simulink model "benchmark_16bus_base_scenario"  (R2021a)
settings: Solver=ode4  StartTime=0.0  StopTime=5  FixedStep=Ts  MaxStep=50e-6  RelTol=1e-3
values from neighbouring files (symbols this model uses):
  Ctrl_Delay = 100e-6    (= 0.0001)    [init_anon.m]
  Pnom1 = 1330e6    (= 1330000000)    [init_anon.m]
  Pnom3 = 1e9    (= 1000000000)    [init_anon.m]
  Pnom4 = 64.4e6    (= 64400000)    [init_anon.m]
  Pnom5 = 19e6    (= 19000000)    [init_anon.m]
  Pnom6 = 450e6    (= 450000000)    [init_anon.m]
  Snom1 = 1e6*sqrt(1330^2 + (0.3*1330)^2)    [init_anon.m]
  Snom3 = 1044e6    (= 1044000000)    [init_anon.m]
  Snom4 = 1e6*sqrt(64.4^2 + (0.3*64.4)^2)    [init_anon.m]
  Snom5 = 1e6*sqrt(19^2 + (0.3*19)^2)    [init_anon.m]
  Snom6 = 1e6*sqrt(450^2 + (0.3*450)^2)    [init_anon.m]
  Ts = 5e-6    (= 5e-06)    [init_anon.m]
  wb = 2*pi*50    (= 314.159265359)    [init_anon.m]
  wcc = 1200    [init_anon.m]
  wlpf = 300    [init_anon.m]
  wp = 10    [init_anon.m]
  wv = 50    [init_anon.m]
  Zb = Ub^2/Sb    [init_anon.m]
undefined symbols (not defined in the file or in its folder): fb, Ib2, Ki_CC, Ki_i, Kp_CC, Kp_i, Kp_Rvi_pu, Lc_eq, Lf_pu, Rc_eq, Sb, Va0, Vb0, Vb1, Vb2, Vc0, Vm0, Vm0_d, Vm0_q, VSC01_id0, Vvsc0
libraries: spsGroundLib x135, spsParallelRLCBranchLib x132, Control_Lib x120, spsSeriesRLCBranchLib x66, spsThreePhaseSourceLib x22, spsThreePhaseBreakerLib x20, eeGeneralControl x20, slpidlib x15, spsLoadFlowBusLib x13, spsThreePhaseVIMeasurementLib x12, spsThreePhaseTransformerTwoWindingsLib x11, spsUniversalBridgeLib x10
(part 5 of 9)

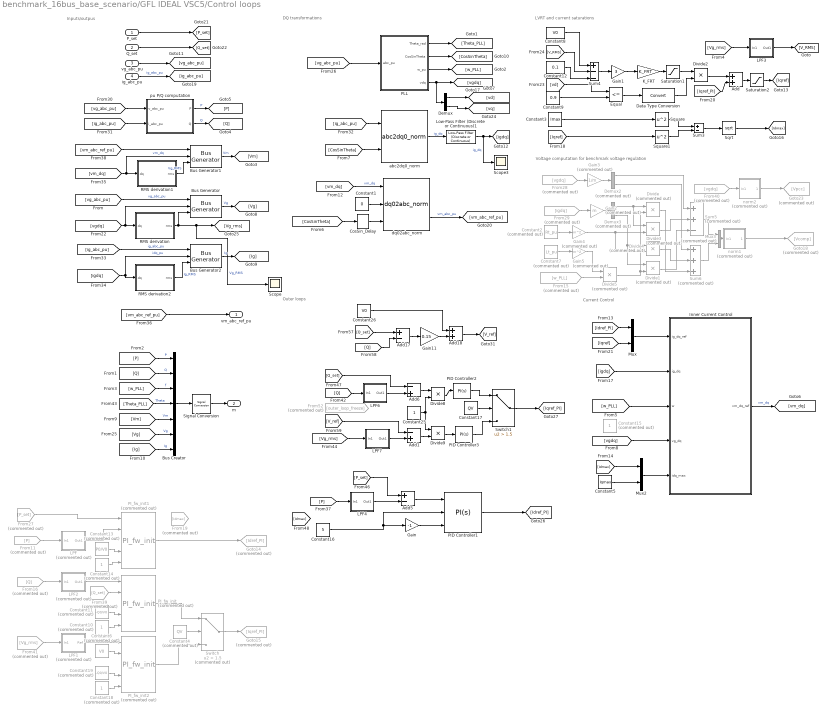
== system benchmark_16bus_base_scenario/GFL IDEAL VSC5/Control loops ==
  note: Inputs/outpus
  note: DQ transformations
  note: Current Control
  note: Outer loops
  note: LVRT and current saturations
  note: Voltage computation for benchmark voltage regulation
  P_set : Inport
  Q_set : Inport  Port=2
  vg_abc_pu : Inport  Port=3
  ig_abc_pu : Inport  Port=4
  " pu P/Q computation" : Subsystem  DialogController=POWERSYS.PowerSysDialog
  Add : Sum
  Add1 : Sum  Inputs=-+
  Add17 : Sum  Inputs=+-
  Add18 : Sum
  Add5 : Sum  Inputs=+-
  Add6 : Sum  Inputs=-+
  Bus Creator : BusCreator  Inputs=7
  Bus Generator : Control_Lib/Bus Generator  Gpu=0
      settings: SourceProductName=VSC4SPS
  Bus Generator1 : Control_Lib/Bus Generator  Gpu=0
      settings: SourceProductName=VSC4SPS
  Bus Generator2 : Control_Lib/Bus Generator  Gpu=0
      settings: SourceProductName=VSC4SPS
  Constant1 : Constant  Value=0
  Constant{10,14..15,18} (4 alike) : Constant  Commented=on
  Constant11 : Constant  Commented=on  Value=-Q0/V0
  Constant12 : Constant  Value=0.1
  Constant13 : Constant  Commented=on  Value=P0/V0
  Constant16 : Constant  Value=5
  Constant17 : Constant  Value=QV
  Constant19 : Constant  Commented=on  Value=-Q0/V0
  Constant2 : Constant  Commented=on  Value=Rt_pu
  Constant25 : Constant
  Constant26 : Constant  Value=V0
  Constant3 : Constant  Value=Imax
  Constant4 : Constant  Commented=on  Value=QV
  Constant5 : Constant  Value=Iqmax
  Constant6 : Constant  Commented=on  Value=V0
  Constant7 : Constant  Commented=on  Value=Lt_pu
  Constant8 : Constant  Value=V0
  Constant9 : Constant  Value=0.9
  CosSin_Delay : Control_Lib/CosSin_Delay  dTheta=wb*Output_Delay
      settings: SourceProductName=VSC4SPS
  Data Type Conversion : DataTypeConversion
  Demux : Demux  Outputs=[1 1]
  Demux2 : Demux  Commented=on  Outputs=2
  Demux3 : Demux  Commented=on  Outputs=2
  Divide{,1,3..5} (5 alike) : Product  Commented=on  Inputs=**
  Divide2 : Product  Inputs=**
  Divide8 : Product  Inputs=**
  Divide9 : Product  Inputs=**
  Equal : RelationalOperator  Operator=<=  OutDataTypeStr=boolean  RndMeth=Simplest
  From11 : From  Commented=on  GotoTag=P
  From15 : From  Commented=on  GotoTag=w_PLL
  From16 : From  Commented=on  GotoTag=Q
  From19 : From  Commented=on  GotoTag=Idmax
  From27 : From  Commented=on  GotoTag=P_set
  From28 : From  Commented=on  GotoTag=vgdq
  From29 : From  Commented=on  GotoTag=igdq
  From39 : From  Commented=on  GotoTag=Q_set
  From40 : From  Commented=on  GotoTag=vgdq
  From41 : From  Commented=on  GotoTag=Vg_rms
  From52 : From  Commented=on  GotoTag=outer_loop_freeze
  Gain : Gain  Gain=-1
  Gain1 : Gain  Gain=3
  Gain11 : Gain  Gain=0.15
  Gain2 : Gain  Commented=on  Gain=m
  Gain3 : Gain  Commented=on  Gain=1/m
  Gain4 : Gain  Commented=on  Gain=m^2
  Gain5 : Gain  Commented=on  Gain=m^2
  Goto14 : Goto  Commented=on  GotoTag=Idref_PI
  Goto15 : Goto  Commented=on  GotoTag=Iqref_PI
  Goto18 : Goto  Commented=on  GotoTag=Vcomp
  Goto23 : Goto  Commented=on  GotoTag=Vpcc
  Inner Current Control : Subsystem
  K_FRT : Gain  Gain=K_FRT
  LPF : Subsystem  Commented=on
  LPF1 : Subsystem  Commented=on
  LPF2 : Subsystem  Commented=on
  LPF3 : Subsystem
  LPF4 : Subsystem
  LPF6 : Subsystem
  LPF7 : Subsystem
  Low-Pass Filter (Discrete or Continuous)1 : eeGeneralControl/Low-Pass Filter (Discrete or Continuous)  K=1  T=1/(2*pi*1e4)  B=inf  A=-inf  init_option=Specify as parameter  x0=[P0/V0 -Q0/V0]  Ts=-1
  Mux : Mux  Inputs=2
  Mux2 : Mux  Inputs=2
  Mux3 : Mux  Commented=on  Inputs=2
  PID Controller1 : slpidlib/PID Controller  Controller=PI  Form=Parallel  TimeDomain=Continuous-time  UseExternalTs=off  SampleTime=-1  IntegratorMethod=Forward Euler  FilterMethod=Forward Euler  ControllerParametersSource=internal  P=w_P/w_LPF  I=w_P  D=0  UseFilter=on  N=100  TunerSelectOption=Transfer Function Based (PID Tuner App)  InitialConditionSource=internal  InitialConditionForIntegrator=P0/V0  InitialConditionForFilter=0  DifferentiatorICPrevScaledInput=0  ExternalReset=none  TrackingMode=off  Kt=1  LimitOutput=on  SatLimitsSource=external  UpperSaturationLimit=inf  LowerSaturationLimit=-inf  LinearizeAsGain=on  AntiWindupMode=clamping  Kb=1  POutMin=[]  POutMax=[]  IOutMin=[]  IOutMax=[]  DOutMin=[]  DOutMax=[]  NOutMin=[]  NOutMax=[]  SumOutMin=[]  SumOutMax=[]  SaturationOutMin=[]  SaturationOutMax=[]  PParamMin=[]  PParamMax=[]  IParamMin=[]  IParamMax=[]  DParamMin=[]  DParamMax=[]  NParamMin=[]  NParamMax=[]  KbParamMin=[]  KbParamMax=[]  KtParamMin=[]  KtParamMax=[]  KbOutMin=[]  KbOutMax=[]  KtOutMin=[]  KtOutMax=[]  IntegratorOutMin=[]  IntegratorOutMax=[]  FilterOutMin=[]  FilterOutMax=[]  SumI1OutMin=[]  SumI1OutMax=[]  SumI2OutMin=[]  SumI2OutMax=[]  SumI3OutMin=[]  SumI3OutMax=[]  SumI4OutMin=[]  SumI4OutMax=[]  SumDOutMin=[]  SumDOutMax=[]  DifferentiatorOutMin=[]  DifferentiatorOutMax=[]  FilterDiffOutCoefMin=[]  FilterDiffOutCoefMax=[]  ReciprocalOutMin=[]  ReciprocalOutMax=[]  SumDenOutMin=[]  SumDenOutMax=[]  SumNumOutMin=[]  SumNumOutMax=[]  DivideOutMin=[]  DivideOutMax=[]  UdiffTsProdOutMin=[]  UdiffTsProdOutMax=[]  NTsProdOutMin=[]  NTsProdOutMax=[]  UintegralTsProdOutMin=[]  UintegralTsProdOutMax=[]  UngainTsProdOutMin=[]  UngainTsProdOutMax=[]  IntegratorContinuousStateAttributes=''  IntegratorStateMustResolveToSignalObject=off  IntegratorRTWStateStorageClass=Auto  FilterContinuousStateAttributes=''  FilterStateMustResolveToSignalObject=off  FilterRTWStateStorageClass=Auto  ParallelPVariant=InternalParameters  IdealPVariant=Disabled  IVariant=InternalParameters  DVariant=Disabled  IntegratorVariant=Continuous  SatVariant=External  AWVariant=ContClampingParallel  PCopyVariant=Disabled  TRVariant=Disabled  FdbkBlocksVariant=Forward  IdealPFdbkVariant=Disabled  SatFdbkVariant=Disabled  DerivativeFilterVariant=Disabled  NVariant=Disabled  NCopyVariant=Disabled_SignalSpec  FilterICVariant=Disabled  IntegratorICVariant=InternalICs  ExternalResetVariant=Disabled  TRSumVariant=Passthrough  SumFdbkVariant=Disabled  SumVariant=Sum_PI  TsampFilterVariant=InternalTs  TsampNgainVariant=Passthrough  TsampIntegralVariant=Passthrough  ExternalSaturationOutDataTypeStr=Inherit: Same as second input
  PID Controller2 : slpidlib/PID Controller  Controller=PI  Form=Parallel  TimeDomain=Continuous-time  UseExternalTs=off  SampleTime=-1  IntegratorMethod=Forward Euler  FilterMethod=Forward Euler  ControllerParametersSource=internal  P=w_P/w_LPF  I=w_P  D=0  UseFilter=on  N=100  TunerSelectOption=Transfer Function Based (PID Tuner App)  InitialConditionSource=internal  InitialConditionForIntegrator=-Q0/V0  InitialConditionForFilter=0  DifferentiatorICPrevScaledInput=0  ExternalReset=none  TrackingMode=off  Kt=1  LimitOutput=on  SatLimitsSource=internal  UpperSaturationLimit=Iqmax*m  LowerSaturationLimit=-Iqmax*m  LinearizeAsGain=on  AntiWindupMode=clamping  Kb=1  POutMin=[]  POutMax=[]  IOutMin=[]  IOutMax=[]  DOutMin=[]  DOutMax=[]  NOutMin=[]  NOutMax=[]  SumOutMin=[]  SumOutMax=[]  SaturationOutMin=[]  SaturationOutMax=[]  PParamMin=[]  PParamMax=[]  IParamMin=[]  IParamMax=[]  DParamMin=[]  DParamMax=[]  NParamMin=[]  NParamMax=[]  KbParamMin=[]  KbParamMax=[]  KtParamMin=[]  KtParamMax=[]  KbOutMin=[]  KbOutMax=[]  KtOutMin=[]  KtOutMax=[]  IntegratorOutMin=[]  IntegratorOutMax=[]  FilterOutMin=[]  FilterOutMax=[]  SumI1OutMin=[]  SumI1OutMax=[]  SumI2OutMin=[]  SumI2OutMax=[]  SumI3OutMin=[]  SumI3OutMax=[]  SumI4OutMin=[]  SumI4OutMax=[]  SumDOutMin=[]  SumDOutMax=[]  DifferentiatorOutMin=[]  DifferentiatorOutMax=[]  FilterDiffOutCoefMin=[]  FilterDiffOutCoefMax=[]  ReciprocalOutMin=[]  ReciprocalOutMax=[]  SumDenOutMin=[]  SumDenOutMax=[]  SumNumOutMin=[]  SumNumOutMax=[]  DivideOutMin=[]  DivideOutMax=[]  UdiffTsProdOutMin=[]  UdiffTsProdOutMax=[]  NTsProdOutMin=[]  NTsProdOutMax=[]  UintegralTsProdOutMin=[]  UintegralTsProdOutMax=[]  UngainTsProdOutMin=[]  UngainTsProdOutMax=[]  IntegratorContinuousStateAttributes=''  IntegratorStateMustResolveToSignalObject=off  IntegratorRTWStateStorageClass=Auto  FilterContinuousStateAttributes=''  FilterStateMustResolveToSignalObject=off  FilterRTWStateStorageClass=Auto  ParallelPVariant=InternalParameters  IdealPVariant=Disabled  IVariant=InternalParameters  DVariant=Disabled  IntegratorVariant=Continuous  SatVariant=Enabled  AWVariant=ContClampingParallel  PCopyVariant=Disabled  TRVariant=Disabled  FdbkBlocksVariant=Forward  IdealPFdbkVariant=Disabled  SatFdbkVariant=Disabled  DerivativeFilterVariant=Disabled  NVariant=Disabled  NCopyVariant=Disabled_SignalSpec  FilterICVariant=Disabled  IntegratorICVariant=InternalICs  ExternalResetVariant=Disabled  TRSumVariant=Passthrough  SumFdbkVariant=Disabled  SumVariant=Sum_PI  TsampFilterVariant=InternalTs  TsampNgainVariant=Passthrough  TsampIntegralVariant=Passthrough  ExternalSaturationOutDataTypeStr=Inherit: Same as second input
  PID Controller3 : slpidlib/PID Controller  Controller=PI  Form=Parallel  TimeDomain=Continuous-time  UseExternalTs=off  SampleTime=-1  IntegratorMethod=Forward Euler  FilterMethod=Forward Euler  ControllerParametersSource=internal  P=w_V/w_LPF  I=w_V  D=0  UseFilter=on  N=100  TunerSelectOption=Transfer Function Based (PID Tuner App)  InitialConditionSource=internal  InitialConditionForIntegrator=-Q0/V0  InitialConditionForFilter=0  DifferentiatorICPrevScaledInput=0  ExternalReset=none  TrackingMode=off  Kt=1  LimitOutput=on  SatLimitsSource=internal  UpperSaturationLimit=Iqmax*m  LowerSaturationLimit=-Iqmax*m  LinearizeAsGain=on  AntiWindupMode=clamping  Kb=1  POutMin=[]  POutMax=[]  IOutMin=[]  IOutMax=[]  DOutMin=[]  DOutMax=[]  NOutMin=[]  NOutMax=[]  SumOutMin=[]  SumOutMax=[]  SaturationOutMin=[]  SaturationOutMax=[]  PParamMin=[]  PParamMax=[]  IParamMin=[]  IParamMax=[]  DParamMin=[]  DParamMax=[]  NParamMin=[]  NParamMax=[]  KbParamMin=[]  KbParamMax=[]  KtParamMin=[]  KtParamMax=[]  KbOutMin=[]  KbOutMax=[]  KtOutMin=[]  KtOutMax=[]  IntegratorOutMin=[]  IntegratorOutMax=[]  FilterOutMin=[]  FilterOutMax=[]  SumI1OutMin=[]  SumI1OutMax=[]  SumI2OutMin=[]  SumI2OutMax=[]  SumI3OutMin=[]  SumI3OutMax=[]  SumI4OutMin=[]  SumI4OutMax=[]  SumDOutMin=[]  SumDOutMax=[]  DifferentiatorOutMin=[]  DifferentiatorOutMax=[]  FilterDiffOutCoefMin=[]  FilterDiffOutCoefMax=[]  ReciprocalOutMin=[]  ReciprocalOutMax=[]  SumDenOutMin=[]  SumDenOutMax=[]  SumNumOutMin=[]  SumNumOutMax=[]  DivideOutMin=[]  DivideOutMax=[]  UdiffTsProdOutMin=[]  UdiffTsProdOutMax=[]  NTsProdOutMin=[]  NTsProdOutMax=[]  UintegralTsProdOutMin=[]  UintegralTsProdOutMax=[]  UngainTsProdOutMin=[]  UngainTsProdOutMax=[]  IntegratorContinuousStateAttributes=''  IntegratorStateMustResolveToSignalObject=off  IntegratorRTWStateStorageClass=Auto  FilterContinuousStateAttributes=''  FilterStateMustResolveToSignalObject=off  FilterRTWStateStorageClass=Auto  ParallelPVariant=InternalParameters  IdealPVariant=Disabled  IVariant=InternalParameters  DVariant=Disabled  IntegratorVariant=Continuous  SatVariant=Enabled  AWVariant=ContClampingParallel  PCopyVariant=Disabled  TRVariant=Disabled  FdbkBlocksVariant=Forward  IdealPFdbkVariant=Disabled  SatFdbkVariant=Disabled  DerivativeFilterVariant=Disabled  NVariant=Disabled  NCopyVariant=Disabled_SignalSpec  FilterICVariant=Disabled  IntegratorICVariant=InternalICs  ExternalResetVariant=Disabled  TRSumVariant=Passthrough  SumFdbkVariant=Disabled  SumVariant=Sum_PI  TsampFilterVariant=InternalTs  TsampNgainVariant=Passthrough  TsampIntegralVariant=Passthrough  ExternalSaturationOutDataTypeStr=Inherit: Same as second input
  PI_fw_init : Control_Lib/PI_fw_init  Commented=on  Kp=w_P/w_LPF  Ki=w_P
      settings: SourceProductName=VSC4SPS
  PI_fw_init1 : Control_Lib/PI_fw_init  Commented=on  Kp=w_P/w_LPF  Ki=w_P
      settings: SourceProductName=VSC4SPS
  PI_fw_init2 : Control_Lib/PI_fw_init  Commented=on  Kp=w_V/w_LPF  Ki=w_V
      settings: SourceProductName=VSC4SPS
  PLL : Subsystem  AncestorBlock=Control_Lib/PLL  TreatAsAtomicUnit=on  mask{fb=fb, wn_PLL=wn_PLL, zeta_PLL=zeta_PLL, Theta0=Theta0}
      mask prompts: fb "fb (Hz)"; wn_PLL "Bandwidth (rad/s)"; zeta_PLL "Damping Ratio"; Theta0 "Theta0 (°)"
      mask init:
      | wb = 2*pi*fb;
      | Kp_PLL = 2*zeta_PLL*wn_PLL/wb;
      | Ki_PLL = wn_PLL^2/wb;
  RMS derivation : Subsystem
  RMS derivation1 : Subsystem
  RMS derivation2 : Subsystem
  Saturation1 : Saturate  UpperLimit=Imax  LowerLimit=-Imax
  Saturation2 : Saturate  UpperLimit=Imax  LowerLimit=-Imax
  Scope : Scope
  Scope3 : Scope
  Signal Conversion : SignalConversion  OverrideOpt=off
  Sqrt : Sqrt  SaturateOnIntegerOverflow=on
  Square : Math  Operator=square  SaturateOnIntegerOverflow=on
  Square1 : Math  Operator=square  SaturateOnIntegerOverflow=on
  Sum3 : Sum  Inputs=+-
  Sum4 : Sum  Inputs=+--
  Sum5 : Sum  Commented=on  Inputs=++-
  Sum6 : Sum  Commented=on  Inputs=+++
  Switch : Switch  Commented=on  Criteria=u2 > Threshold  Threshold=1.5
  Switch1 : Switch  Criteria=u2 > Threshold  Threshold=1.5
  abc2dq0_norm : Control_Lib/abc2dq0_norm  referenceAxisMode=Reference axis at 90 degrees behind phase_a  baseUpdateGain=1/sqrt(3)
      settings: SourceProductName=VSC4SPS
  dq02abc_norm : Control_Lib/dq02abc_norm  referenceAxisMode=Reference axis at 90 degrees behind phase_a  baseUpdateGain=sqrt(3)
      settings: SourceProductName=VSC4SPS
  norm1 : Subsystem  Commented=on
  norm2 : Subsystem  Commented=on
  vm_abc_ref_pu : Outport  VectorParamsAs1DForOutWhenUnconnected=off
  m : Outport  Port=2  VectorParamsAs1DForOutWhenUnconnected=off
  wires:
  Low-Pass Filter (Discrete or Continuous)1/1 -> Scope3/1, [igdq]  "ig_dq"
  [Q_set] -> Add6/1
  [P_set] -> Add5/1
  Switch1/1 -> [Iqref_PI]
  Gain/1 -> PID Controller1/3
  PID Controller3/1 -> Switch1/3
  [Vg_rms] -> LPF7/1(In1)
  PID Controller2/1 -> Switch1/1
  [Q] -> LPF6/1(In1)
  Constant17/1 -> Switch1/2
  Add5/1 -> PID Controller1/1
  LPF4/1(Out1) -> Add5/2
  [P] -> LPF4/1(In1)
  LPF6/1(Out1) -> Add6/2
  PID Controller1/1 -> [Idref_PI]
  Add6/1 -> Divide8/1
  Divide8/1 -> PID Controller2/1
  Divide9/1 -> PID Controller3/1
  Add1/1 -> Divide9/2
  Constant25/1 -> Divide9/1, Divide8/2
  Constant16/1 -> Gain/1, PID Controller1/2
  LPF7/1(Out1) -> Add1/2
  [V_ref] -> Add1/1
  [Q] -> Add17/2
  Constant26/1 -> Add18/1
  [Q_set] -> Add17/1
  Gain11/1 -> Add18/2
  Add17/1 -> Gain11/1
  Add18/1 -> [V_ref]
  [w_PLL] -> Inner Current Control/3(w)
  Constant6/1 -> PI_fw_init2/2
  PI_fw_init2/1 -> Switch/3
  Constant14/1 -> PI_fw_init1/5
  Constant13/1 -> PI_fw_init1/4
  [Vg_rms] -> LPF3/1(In1)
  LPF3/1(Out1) -> [V_RMS]
  CosSin_Delay/1 -> dq02abc_norm/3
  [Theta_PLL] -> Bus Creator/4  "Theta"
  RMS derivation/1(rms) -> Bus Generator/3, [Vg_rms], Scope/1  "Vg_RMS"
  [vgdq] -> Bus Generator/2, RMS derivation/1(dq)
  Demux/2 -> [vq]
  Demux/1 -> [vd]
  PLL/4(vdq) -> [vgdq], Demux/1
  norm2/1(Out1) -> Goto23/1
  From40/1 -> norm2/1(In1)
  Gain4/1 -> Divide3/2, Divide4/2
  Gain5/1 -> Divide5/1
  Gain2/1 -> Demux3/1
  From29/1 -> Gain2/1
  From39/1 -> PI_fw_init/2
  [vgdq] -> Inner Current Control/4(vg_dq)
  [vm_abc_ref_pu] -> Bus Generator1/1
  [vm_abc_ref_pu] -> vm_abc_ref_pu/1
  [vm_dq] -> Bus Generator1/2, RMS derivation1/1(dq)  "vm_dq"
  [ig_abc_pu] -> abc2dq0_norm/1
  [ig_abc_pu] -> " pu P/Q computation"/2(i_abc_pu)
  [vg_abc_pu] -> " pu P/Q computation"/1(v_abc_pu)
  [vg_abc_pu] -> PLL/1(abc_pu)
  From41/1 -> LPF1/1(In1)
  Constant7/1 -> Gain5/1
  From15/1 -> Divide5/2
  PLL/3(w_pu) -> [w_PLL]
  PLL/2(CosSinTheta) -> [CosSinTheta]
  PLL/1(Theta_rad) -> [Theta_PLL]
  Demux3/1 -> Divide3/1, Divide/1
  Divide4/1 -> Sum6/2
  Demux3/2 -> Divide4/1, Divide1/1
  Divide3/1 -> Sum5/2
  Demux2/1 -> Sum5/1
  Divide5/1 -> Divide1/2, Divide/2
  Divide/1 -> Sum6/3
  Mux3/1 -> norm1/1(In1)
  Sum6/1 -> Mux3/2
  Divide1/1 -> Sum5/3
  norm1/1(Out1) -> Goto18/1
  Constant2/1 -> Gain4/1
  Gain3/1 -> Demux2/1
  Demux2/2 -> Sum6/1
  From28/1 -> Gain3/1
  Sum5/1 -> Mux3/1
  Gain1/1 -> K_FRT/1
  [Iqref] -> Square1/1
  Square/1 -> Sum3/1
  Constant3/1 -> Square/1
  Sum3/1 -> Sqrt/1
  Sqrt/1 -> [Idmax]
  Square1/1 -> Sum3/2
  LPF1/1(Ref) -> PI_fw_init2/1
  Q_set/1 -> [Q_set]
  From16/1 -> LPF2/1(In1)
  [Idmax] -> Mux2/1
  Constant5/1 -> Mux2/2
  Mux2/1 -> Inner Current Control/5(idq_max)
  [Iqref_PI] -> Add/2
  Add/1 -> Saturation2/1
  Constant4/1 -> Switch/2
  Constant9/1 -> Equal/2
  Constant8/1 -> Sum4/1
  Constant12/1 -> Sum4/3
  Divide2/1 -> Add/1
  [vd] -> Equal/1
  Data Type Conversion/1 -> Divide2/2
  Equal/1 -> Data Type Conversion/1
  Saturation1/1 -> Divide2/1
  K_FRT/1 -> Saturation1/1
  [V_RMS] -> Sum4/2
  Sum4/1 -> Gain1/1
  Saturation2/1 -> [Iqref]
  [igdq] -> Inner Current Control/2(ig_dq)
  [Idref_PI] -> Mux/1
  [Iqref] -> Mux/2
  From11/1 -> LPF/1(In1)
  P_set/1 -> [P_set]
  Bus Creator/1 -> Signal Conversion/1
  Bus Generator/1 -> [Vg]  "Vg"
  [CosSinTheta] -> abc2dq0_norm/2
  [CosSinTheta] -> CosSin_Delay/1
  abc2dq0_norm/2 -> Low-Pass Filter (Discrete or Continuous)1/1  "ig_dq"
  ig_abc_pu/1 -> [ig_abc_pu]  "ig_abc_pu"
  " pu P/Q computation"/1(P) -> [P]  "P"
  vg_abc_pu/1 -> [vg_abc_pu]
  Inner Current Control/1(vm_dq_ref) -> [vm_dq]  "vm_dq"
  [vm_dq] -> dq02abc_norm/1  "vm_dq"
  " pu P/Q computation"/2(Q) -> [Q]  "Q"
  dq02abc_norm/2 -> [vm_abc_ref_pu]  "vm_abc_pu"
  [w_PLL] -> Bus Creator/3  "f"
  [Q] -> Bus Creator/2  "Q"
  [P] -> Bus Creator/1  "P"
  Signal Conversion/1 -> m/1
  Mux/1 -> Inner Current Control/1(ig_dq_ref)
  Constant1/1 -> dq02abc_norm/2
  [vg_abc_pu] -> Bus Generator/1  "vg_abc_pu"
  RMS derivation1/1(rms) -> Bus Generator1/3  "Vg_RMS"
  Bus Generator1/1 -> [Vm]  "Vm"
  [Vm] -> Bus Creator/5  "Vm"
  [Vg] -> Bus Creator/6  "Vg"
  [Ig] -> Bus Creator/7  "Ig"
  [ig_abc_pu] -> Bus Generator2/1  "ig_abc_pu"
  Bus Generator2/1 -> [Ig]  "Ig"
  [igdq] -> RMS derivation2/1(dq), Bus Generator2/2  "idq_pu"
  RMS derivation2/1(rms) -> Bus Generator2/3  "Ig_RMS"
  Constant11/1 -> PI_fw_init/4
  Constant10/1 -> PI_fw_init/5
  PI_fw_init/1 -> Switch/1
  LPF2/1(Out1) -> PI_fw_init/1
  Constant18/1 -> PI_fw_init2/5
  Constant19/1 -> PI_fw_init2/4
  Switch/1 -> Goto15/1
  LPF/1(Out1) -> PI_fw_init1/2
  From27/1 -> PI_fw_init1/1
  PI_fw_init1/1 -> Goto14/1

== system benchmark_16bus_base_scenario/GFL IDEAL VSC6/Bridge_Model ==
  Uref : Inport
  NOT1 : Logic  Operator=NOT  IconShape=distinctive  AllPortsSameDT=off  OutDataTypeStr=boolean
  Saturation : Saturate  UpperLimit=1  LowerLimit=-1
  Step : Step  Time=Output_Delay  SampleTime=0
  Terminator : Terminator
  Three-Phase Breaker2 : spsThreePhaseBreakerLib/Three-Phase Breaker  InitialState=open  SwitchA=on  SwitchB=on  SwitchC=on  SwitchTimes="[4/60  10/60]"  External=on  BreakerResistance=1e-5*Zb  SnubberResistance=1e6  SnubberCapacitance=inf  Measurements=None
  Three-Phase Breaker3 : spsThreePhaseBreakerLib/Three-Phase Breaker  InitialState=closed  SwitchA=on  SwitchB=on  SwitchC=on  SwitchTimes="[4/60  10/60]"  External=on  BreakerResistance=1e-6*Zb  SnubberResistance=1e6  SnubberCapacitance=inf  Measurements=None
  Three-Phase Source : spsThreePhaseSourceLib/Three-Phase Source  InternalConnection=Yg  VoltagePhases=off  Voltage=Vm0*Un1  PhaseAngle=Theta_Vm0  Voltage_phases=[25e3 25e3 25e3]/sqrt(3)  PhaseAngles_phases=[0 -120 +120]  Frequency=fb  NonIdealSource=off  SpecifyImpedance=off  Resistance=0  Inductance=0  ShortCircuitLevel=100e6  BaseVoltage=VSC01_Un1  XRratio=7  BusType=swing  Pref=0.3  Qref=0  Prefabc=[10e3, 10e3, 10e3]  Qrefabc=[0, 0, 0]  Qmin=-Inf  Qmax=Inf
  Universal Bridge : spsUniversalBridgeLib/Universal Bridge  Arms=3  SnubberResistance=1e5  SnubberCapacitance=inf  Device=Average-model based VSC  Ron=1e-3  Lon=0  ForwardVoltages="[  0  0  ]"  ForwardVoltage=0  GTOparameters=[ 10e-6 , 20e-6 ]  IGBTparameters=[ 1e-6 , 2e-6 ]  Measurements=None  Measurements_2=None  converterType=Rectifier
  Vdc : spsVoltageMeasurementLib/Voltage Measurement  PhasorSimulation=off  OutputType=Complex  PSBequivalent=0
  mp3 : Gain  Gain=2/Udcn
  PhA : PMIOPort  Side=Right
  PhB : PMIOPort  Port=2  Side=Right
  PhC : PMIOPort  Port=3  Side=Right
  Vdc+ : PMIOPort  Port=4  Side=Left
  Vdc- : PMIOPort  Port=5  Side=Left
  wires:
  Vdc/1 -> Terminator/1
  Uref/1 -> mp3/1
  mp3/1 -> Saturation/1
  NOT1/1 -> Three-Phase Breaker3/1
  Saturation/1 -> Universal Bridge/1
  Step/1 -> NOT1/1, Three-Phase Breaker2/1
  connections:
  Vdc-/RConn1 -- Universal Bridge/RConn2 -- Vdc/LConn2
  Vdc+/RConn1 -- Universal Bridge/RConn1 -- Vdc/LConn1
  PhC/RConn1 -- Three-Phase Breaker3/LConn3 -- Three-Phase Breaker2/LConn3
  PhB/RConn1 -- Three-Phase Breaker3/LConn2 -- Three-Phase Breaker2/LConn2
  PhA/RConn1 -- Three-Phase Breaker3/LConn1 -- Three-Phase Breaker2/LConn1
  Three-Phase Breaker2/RConn3 -- Universal Bridge/LConn3
  Three-Phase Breaker2/RConn2 -- Universal Bridge/LConn2
  Three-Phase Breaker2/RConn1 -- Universal Bridge/LConn1
  Three-Phase Breaker3/RConn1 -- Three-Phase Source/RConn1
  Three-Phase Breaker3/RConn2 -- Three-Phase Source/RConn2
  Three-Phase Breaker3/RConn3 -- Three-Phase Source/RConn3

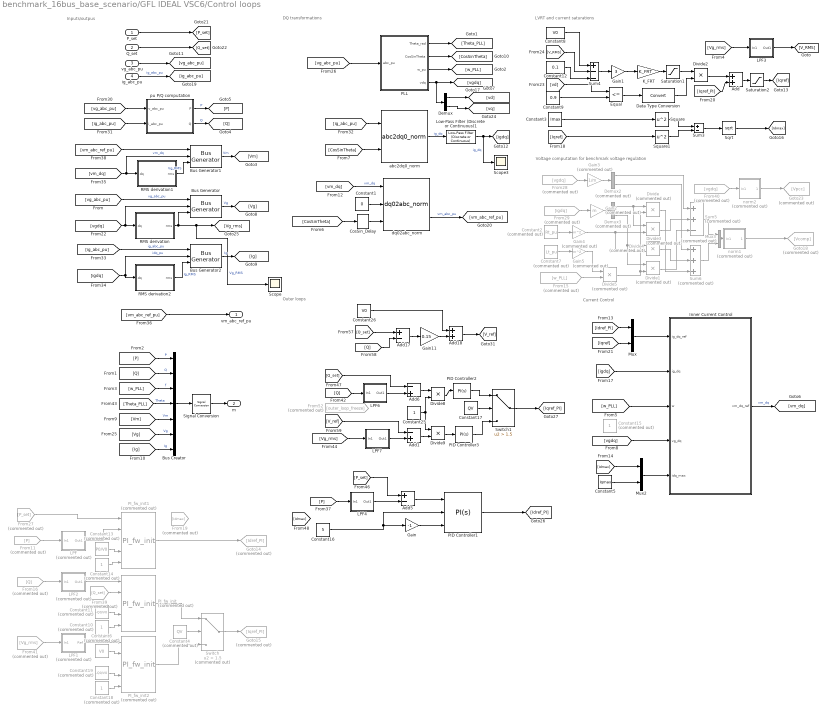
== system benchmark_16bus_base_scenario/GFL IDEAL VSC6/Control loops ==
  note: Voltage computation for benchmark voltage regulation
  note: LVRT and current saturations
  note: Outer loops
  note: Current Control
  note: DQ transformations
  note: Inputs/outpus
  P_set : Inport
  Q_set : Inport  Port=2
  vg_abc_pu : Inport  Port=3
  ig_abc_pu : Inport  Port=4
  " pu P/Q computation" : Subsystem  DialogController=POWERSYS.PowerSysDialog
  Add : Sum
  Add1 : Sum  Inputs=-+
  Add17 : Sum  Inputs=+-
  Add18 : Sum
  Add5 : Sum  Inputs=+-
  Add6 : Sum  Inputs=-+
  Bus Creator : BusCreator  Inputs=7
  Bus Generator : Control_Lib/Bus Generator  Gpu=0
      settings: SourceProductName=VSC4SPS
  Bus Generator1 : Control_Lib/Bus Generator  Gpu=0
      settings: SourceProductName=VSC4SPS
  Bus Generator2 : Control_Lib/Bus Generator  Gpu=0
      settings: SourceProductName=VSC4SPS
  Constant1 : Constant  Value=0
  Constant{10,14..15,18} (4 alike) : Constant  Commented=on
  Constant11 : Constant  Commented=on  Value=-Q0/V0
  Constant12 : Constant  Value=0.1
  Constant13 : Constant  Commented=on  Value=P0/V0
  Constant16 : Constant  Value=5
  Constant17 : Constant  Value=QV
  Constant19 : Constant  Commented=on  Value=-Q0/V0
  Constant2 : Constant  Commented=on  Value=Rt_pu
  Constant25 : Constant
  Constant26 : Constant  Value=V0
  Constant3 : Constant  Value=Imax
  Constant4 : Constant  Commented=on  Value=QV
  Constant5 : Constant  Value=Iqmax
  Constant6 : Constant  Commented=on  Value=V0
  Constant7 : Constant  Commented=on  Value=Lt_pu
  Constant8 : Constant  Value=V0
  Constant9 : Constant  Value=0.9
  CosSin_Delay : Control_Lib/CosSin_Delay  dTheta=wb*Output_Delay
      settings: SourceProductName=VSC4SPS
  Data Type Conversion : DataTypeConversion
  Demux : Demux  Outputs=[1 1]
  Demux2 : Demux  Commented=on  Outputs=2
  Demux3 : Demux  Commented=on  Outputs=2
  Divide{,1,3..5} (5 alike) : Product  Commented=on  Inputs=**
  Divide2 : Product  Inputs=**
  Divide8 : Product  Inputs=**
  Divide9 : Product  Inputs=**
  Equal : RelationalOperator  Operator=<=  OutDataTypeStr=boolean  RndMeth=Simplest
  From11 : From  Commented=on  GotoTag=P
  From15 : From  Commented=on  GotoTag=w_PLL
  From16 : From  Commented=on  GotoTag=Q
  From19 : From  Commented=on  GotoTag=Idmax
  From27 : From  Commented=on  GotoTag=P_set
  From28 : From  Commented=on  GotoTag=vgdq
  From29 : From  Commented=on  GotoTag=igdq
  From39 : From  Commented=on  GotoTag=Q_set
  From40 : From  Commented=on  GotoTag=vgdq
  From41 : From  Commented=on  GotoTag=Vg_rms
  From52 : From  Commented=on  GotoTag=outer_loop_freeze
  Gain : Gain  Gain=-1
  Gain1 : Gain  Gain=3
  Gain11 : Gain  Gain=0.15
  Gain2 : Gain  Commented=on  Gain=m
  Gain3 : Gain  Commented=on  Gain=1/m
  Gain4 : Gain  Commented=on  Gain=m^2
  Gain5 : Gain  Commented=on  Gain=m^2
  Goto14 : Goto  Commented=on  GotoTag=Idref_PI
  Goto15 : Goto  Commented=on  GotoTag=Iqref_PI
  Goto18 : Goto  Commented=on  GotoTag=Vcomp
  Goto23 : Goto  Commented=on  GotoTag=Vpcc
  Inner Current Control : Subsystem
  K_FRT : Gain  Gain=K_FRT
  LPF : Subsystem  Commented=on
  LPF1 : Subsystem  Commented=on
  LPF2 : Subsystem  Commented=on
  LPF3 : Subsystem
  LPF4 : Subsystem
  LPF6 : Subsystem
  LPF7 : Subsystem
  Low-Pass Filter (Discrete or Continuous)1 : eeGeneralControl/Low-Pass Filter (Discrete or Continuous)  K=1  T=1/(2*pi*1e4)  B=inf  A=-inf  init_option=Specify as parameter  x0=[P0/V0 -Q0/V0]  Ts=-1
  Mux : Mux  Inputs=2
  Mux2 : Mux  Inputs=2
  Mux3 : Mux  Commented=on  Inputs=2
  PID Controller1 : slpidlib/PID Controller  Controller=PI  Form=Parallel  TimeDomain=Continuous-time  UseExternalTs=off  SampleTime=-1  IntegratorMethod=Forward Euler  FilterMethod=Forward Euler  ControllerParametersSource=internal  P=w_P/w_LPF  I=w_P  D=0  UseFilter=on  N=100  TunerSelectOption=Transfer Function Based (PID Tuner App)  InitialConditionSource=internal  InitialConditionForIntegrator=P0/V0  InitialConditionForFilter=0  DifferentiatorICPrevScaledInput=0  ExternalReset=none  TrackingMode=off  Kt=1  LimitOutput=on  SatLimitsSource=external  UpperSaturationLimit=inf  LowerSaturationLimit=-inf  LinearizeAsGain=on  AntiWindupMode=clamping  Kb=1  POutMin=[]  POutMax=[]  IOutMin=[]  IOutMax=[]  DOutMin=[]  DOutMax=[]  NOutMin=[]  NOutMax=[]  SumOutMin=[]  SumOutMax=[]  SaturationOutMin=[]  SaturationOutMax=[]  PParamMin=[]  PParamMax=[]  IParamMin=[]  IParamMax=[]  DParamMin=[]  DParamMax=[]  NParamMin=[]  NParamMax=[]  KbParamMin=[]  KbParamMax=[]  KtParamMin=[]  KtParamMax=[]  KbOutMin=[]  KbOutMax=[]  KtOutMin=[]  KtOutMax=[]  IntegratorOutMin=[]  IntegratorOutMax=[]  FilterOutMin=[]  FilterOutMax=[]  SumI1OutMin=[]  SumI1OutMax=[]  SumI2OutMin=[]  SumI2OutMax=[]  SumI3OutMin=[]  SumI3OutMax=[]  SumI4OutMin=[]  SumI4OutMax=[]  SumDOutMin=[]  SumDOutMax=[]  DifferentiatorOutMin=[]  DifferentiatorOutMax=[]  FilterDiffOutCoefMin=[]  FilterDiffOutCoefMax=[]  ReciprocalOutMin=[]  ReciprocalOutMax=[]  SumDenOutMin=[]  SumDenOutMax=[]  SumNumOutMin=[]  SumNumOutMax=[]  DivideOutMin=[]  DivideOutMax=[]  UdiffTsProdOutMin=[]  UdiffTsProdOutMax=[]  NTsProdOutMin=[]  NTsProdOutMax=[]  UintegralTsProdOutMin=[]  UintegralTsProdOutMax=[]  UngainTsProdOutMin=[]  UngainTsProdOutMax=[]  IntegratorContinuousStateAttributes=''  IntegratorStateMustResolveToSignalObject=off  IntegratorRTWStateStorageClass=Auto  FilterContinuousStateAttributes=''  FilterStateMustResolveToSignalObject=off  FilterRTWStateStorageClass=Auto  ParallelPVariant=InternalParameters  IdealPVariant=Disabled  IVariant=InternalParameters  DVariant=Disabled  IntegratorVariant=Continuous  SatVariant=External  AWVariant=ContClampingParallel  PCopyVariant=Disabled  TRVariant=Disabled  FdbkBlocksVariant=Forward  IdealPFdbkVariant=Disabled  SatFdbkVariant=Disabled  DerivativeFilterVariant=Disabled  NVariant=Disabled  NCopyVariant=Disabled_SignalSpec  FilterICVariant=Disabled  IntegratorICVariant=InternalICs  ExternalResetVariant=Disabled  TRSumVariant=Passthrough  SumFdbkVariant=Disabled  SumVariant=Sum_PI  TsampFilterVariant=InternalTs  TsampNgainVariant=Passthrough  TsampIntegralVariant=Passthrough  ExternalSaturationOutDataTypeStr=Inherit: Same as second input
  PID Controller2 : slpidlib/PID Controller  Controller=PI  Form=Parallel  TimeDomain=Continuous-time  UseExternalTs=off  SampleTime=-1  IntegratorMethod=Forward Euler  FilterMethod=Forward Euler  ControllerParametersSource=internal  P=w_P/w_LPF  I=w_P  D=0  UseFilter=on  N=100  TunerSelectOption=Transfer Function Based (PID Tuner App)  InitialConditionSource=internal  InitialConditionForIntegrator=-Q0/V0  InitialConditionForFilter=0  DifferentiatorICPrevScaledInput=0  ExternalReset=none  TrackingMode=off  Kt=1  LimitOutput=on  SatLimitsSource=internal  UpperSaturationLimit=Iqmax*m  LowerSaturationLimit=-Iqmax*m  LinearizeAsGain=on  AntiWindupMode=clamping  Kb=1  POutMin=[]  POutMax=[]  IOutMin=[]  IOutMax=[]  DOutMin=[]  DOutMax=[]  NOutMin=[]  NOutMax=[]  SumOutMin=[]  SumOutMax=[]  SaturationOutMin=[]  SaturationOutMax=[]  PParamMin=[]  PParamMax=[]  IParamMin=[]  IParamMax=[]  DParamMin=[]  DParamMax=[]  NParamMin=[]  NParamMax=[]  KbParamMin=[]  KbParamMax=[]  KtParamMin=[]  KtParamMax=[]  KbOutMin=[]  KbOutMax=[]  KtOutMin=[]  KtOutMax=[]  IntegratorOutMin=[]  IntegratorOutMax=[]  FilterOutMin=[]  FilterOutMax=[]  SumI1OutMin=[]  SumI1OutMax=[]  SumI2OutMin=[]  SumI2OutMax=[]  SumI3OutMin=[]  SumI3OutMax=[]  SumI4OutMin=[]  SumI4OutMax=[]  SumDOutMin=[]  SumDOutMax=[]  DifferentiatorOutMin=[]  DifferentiatorOutMax=[]  FilterDiffOutCoefMin=[]  FilterDiffOutCoefMax=[]  ReciprocalOutMin=[]  ReciprocalOutMax=[]  SumDenOutMin=[]  SumDenOutMax=[]  SumNumOutMin=[]  SumNumOutMax=[]  DivideOutMin=[]  DivideOutMax=[]  UdiffTsProdOutMin=[]  UdiffTsProdOutMax=[]  NTsProdOutMin=[]  NTsProdOutMax=[]  UintegralTsProdOutMin=[]  UintegralTsProdOutMax=[]  UngainTsProdOutMin=[]  UngainTsProdOutMax=[]  IntegratorContinuousStateAttributes=''  IntegratorStateMustResolveToSignalObject=off  IntegratorRTWStateStorageClass=Auto  FilterContinuousStateAttributes=''  FilterStateMustResolveToSignalObject=off  FilterRTWStateStorageClass=Auto  ParallelPVariant=InternalParameters  IdealPVariant=Disabled  IVariant=InternalParameters  DVariant=Disabled  IntegratorVariant=Continuous  SatVariant=Enabled  AWVariant=ContClampingParallel  PCopyVariant=Disabled  TRVariant=Disabled  FdbkBlocksVariant=Forward  IdealPFdbkVariant=Disabled  SatFdbkVariant=Disabled  DerivativeFilterVariant=Disabled  NVariant=Disabled  NCopyVariant=Disabled_SignalSpec  FilterICVariant=Disabled  IntegratorICVariant=InternalICs  ExternalResetVariant=Disabled  TRSumVariant=Passthrough  SumFdbkVariant=Disabled  SumVariant=Sum_PI  TsampFilterVariant=InternalTs  TsampNgainVariant=Passthrough  TsampIntegralVariant=Passthrough  ExternalSaturationOutDataTypeStr=Inherit: Same as second input
  PID Controller3 : slpidlib/PID Controller  Controller=PI  Form=Parallel  TimeDomain=Continuous-time  UseExternalTs=off  SampleTime=-1  IntegratorMethod=Forward Euler  FilterMethod=Forward Euler  ControllerParametersSource=internal  P=w_V/w_LPF  I=w_V  D=0  UseFilter=on  N=100  TunerSelectOption=Transfer Function Based (PID Tuner App)  InitialConditionSource=internal  InitialConditionForIntegrator=-Q0/V0  InitialConditionForFilter=0  DifferentiatorICPrevScaledInput=0  ExternalReset=none  TrackingMode=off  Kt=1  LimitOutput=on  SatLimitsSource=internal  UpperSaturationLimit=Iqmax*m  LowerSaturationLimit=-Iqmax*m  LinearizeAsGain=on  AntiWindupMode=clamping  Kb=1  POutMin=[]  POutMax=[]  IOutMin=[]  IOutMax=[]  DOutMin=[]  DOutMax=[]  NOutMin=[]  NOutMax=[]  SumOutMin=[]  SumOutMax=[]  SaturationOutMin=[]  SaturationOutMax=[]  PParamMin=[]  PParamMax=[]  IParamMin=[]  IParamMax=[]  DParamMin=[]  DParamMax=[]  NParamMin=[]  NParamMax=[]  KbParamMin=[]  KbParamMax=[]  KtParamMin=[]  KtParamMax=[]  KbOutMin=[]  KbOutMax=[]  KtOutMin=[]  KtOutMax=[]  IntegratorOutMin=[]  IntegratorOutMax=[]  FilterOutMin=[]  FilterOutMax=[]  SumI1OutMin=[]  SumI1OutMax=[]  SumI2OutMin=[]  SumI2OutMax=[]  SumI3OutMin=[]  SumI3OutMax=[]  SumI4OutMin=[]  SumI4OutMax=[]  SumDOutMin=[]  SumDOutMax=[]  DifferentiatorOutMin=[]  DifferentiatorOutMax=[]  FilterDiffOutCoefMin=[]  FilterDiffOutCoefMax=[]  ReciprocalOutMin=[]  ReciprocalOutMax=[]  SumDenOutMin=[]  SumDenOutMax=[]  SumNumOutMin=[]  SumNumOutMax=[]  DivideOutMin=[]  DivideOutMax=[]  UdiffTsProdOutMin=[]  UdiffTsProdOutMax=[]  NTsProdOutMin=[]  NTsProdOutMax=[]  UintegralTsProdOutMin=[]  UintegralTsProdOutMax=[]  UngainTsProdOutMin=[]  UngainTsProdOutMax=[]  IntegratorContinuousStateAttributes=''  IntegratorStateMustResolveToSignalObject=off  IntegratorRTWStateStorageClass=Auto  FilterContinuousStateAttributes=''  FilterStateMustResolveToSignalObject=off  FilterRTWStateStorageClass=Auto  ParallelPVariant=InternalParameters  IdealPVariant=Disabled  IVariant=InternalParameters  DVariant=Disabled  IntegratorVariant=Continuous  SatVariant=Enabled  AWVariant=ContClampingParallel  PCopyVariant=Disabled  TRVariant=Disabled  FdbkBlocksVariant=Forward  IdealPFdbkVariant=Disabled  SatFdbkVariant=Disabled  DerivativeFilterVariant=Disabled  NVariant=Disabled  NCopyVariant=Disabled_SignalSpec  FilterICVariant=Disabled  IntegratorICVariant=InternalICs  ExternalResetVariant=Disabled  TRSumVariant=Passthrough  SumFdbkVariant=Disabled  SumVariant=Sum_PI  TsampFilterVariant=InternalTs  TsampNgainVariant=Passthrough  TsampIntegralVariant=Passthrough  ExternalSaturationOutDataTypeStr=Inherit: Same as second input
  PI_fw_init : Control_Lib/PI_fw_init  Commented=on  Kp=w_P/w_LPF  Ki=w_P
      settings: SourceProductName=VSC4SPS
  PI_fw_init1 : Control_Lib/PI_fw_init  Commented=on  Kp=w_P/w_LPF  Ki=w_P
      settings: SourceProductName=VSC4SPS
  PI_fw_init2 : Control_Lib/PI_fw_init  Commented=on  Kp=w_V/w_LPF  Ki=w_V
      settings: SourceProductName=VSC4SPS
  PLL : Subsystem  AncestorBlock=Control_Lib/PLL  TreatAsAtomicUnit=on  mask{fb=fb, wn_PLL=wn_PLL, zeta_PLL=zeta_PLL, Theta0=Theta0}
      mask prompts: fb "fb (Hz)"; wn_PLL "Bandwidth (rad/s)"; zeta_PLL "Damping Ratio"; Theta0 "Theta0 (°)"
      mask init:
      | wb = 2*pi*fb;
      | Kp_PLL = 2*zeta_PLL*wn_PLL/wb;
      | Ki_PLL = wn_PLL^2/wb;
  RMS derivation : Subsystem
  RMS derivation1 : Subsystem
  RMS derivation2 : Subsystem
  Saturation1 : Saturate  UpperLimit=Imax  LowerLimit=-Imax
  Saturation2 : Saturate  UpperLimit=Imax  LowerLimit=-Imax
  Scope : Scope
  Scope3 : Scope
  Signal Conversion : SignalConversion  OverrideOpt=off
  Sqrt : Sqrt  SaturateOnIntegerOverflow=on
  Square : Math  Operator=square  SaturateOnIntegerOverflow=on
  Square1 : Math  Operator=square  SaturateOnIntegerOverflow=on
  Sum3 : Sum  Inputs=+-
  Sum4 : Sum  Inputs=+--
  Sum5 : Sum  Commented=on  Inputs=++-
  Sum6 : Sum  Commented=on  Inputs=+++
  Switch : Switch  Commented=on  Criteria=u2 > Threshold  Threshold=1.5
  Switch1 : Switch  Criteria=u2 > Threshold  Threshold=1.5
  abc2dq0_norm : Control_Lib/abc2dq0_norm  referenceAxisMode=Reference axis at 90 degrees behind phase_a  baseUpdateGain=1/sqrt(3)
      settings: SourceProductName=VSC4SPS
  dq02abc_norm : Control_Lib/dq02abc_norm  referenceAxisMode=Reference axis at 90 degrees behind phase_a  baseUpdateGain=sqrt(3)
      settings: SourceProductName=VSC4SPS
  norm1 : Subsystem  Commented=on
  norm2 : Subsystem  Commented=on
  vm_abc_ref_pu : Outport  VectorParamsAs1DForOutWhenUnconnected=off
  m : Outport  Port=2  VectorParamsAs1DForOutWhenUnconnected=off
  wires:
  PI_fw_init1/1 -> Goto14/1
  From27/1 -> PI_fw_init1/1
  LPF/1(Out1) -> PI_fw_init1/2
  Switch/1 -> Goto15/1
  Constant19/1 -> PI_fw_init2/4
  Constant18/1 -> PI_fw_init2/5
  LPF2/1(Out1) -> PI_fw_init/1
  PI_fw_init/1 -> Switch/1
  Constant10/1 -> PI_fw_init/5
  Constant11/1 -> PI_fw_init/4
  RMS derivation2/1(rms) -> Bus Generator2/3  "Ig_RMS"
  [igdq] -> Bus Generator2/2, RMS derivation2/1(dq)  "idq_pu"
  Bus Generator2/1 -> [Ig]  "Ig"
  [ig_abc_pu] -> Bus Generator2/1  "ig_abc_pu"
  [Ig] -> Bus Creator/7  "Ig"
  [Vg] -> Bus Creator/6  "Vg"
  [Vm] -> Bus Creator/5  "Vm"
  Bus Generator1/1 -> [Vm]  "Vm"
  RMS derivation1/1(rms) -> Bus Generator1/3  "Vg_RMS"
  [vg_abc_pu] -> Bus Generator/1  "vg_abc_pu"
  Constant1/1 -> dq02abc_norm/2
  Mux/1 -> Inner Current Control/1(ig_dq_ref)
  Signal Conversion/1 -> m/1
  [P] -> Bus Creator/1  "P"
  [Q] -> Bus Creator/2  "Q"
  [w_PLL] -> Bus Creator/3  "f"
  dq02abc_norm/2 -> [vm_abc_ref_pu]  "vm_abc_pu"
  " pu P/Q computation"/2(Q) -> [Q]  "Q"
  [vm_dq] -> dq02abc_norm/1  "vm_dq"
  Inner Current Control/1(vm_dq_ref) -> [vm_dq]  "vm_dq"
  vg_abc_pu/1 -> [vg_abc_pu]
  " pu P/Q computation"/1(P) -> [P]  "P"
  ig_abc_pu/1 -> [ig_abc_pu]  "ig_abc_pu"
  abc2dq0_norm/2 -> Low-Pass Filter (Discrete or Continuous)1/1  "ig_dq"
  [CosSinTheta] -> CosSin_Delay/1
  [CosSinTheta] -> abc2dq0_norm/2
  Bus Generator/1 -> [Vg]  "Vg"
  Bus Creator/1 -> Signal Conversion/1
  P_set/1 -> [P_set]
  From11/1 -> LPF/1(In1)
  [Iqref] -> Mux/2
  [Idref_PI] -> Mux/1
  [igdq] -> Inner Current Control/2(ig_dq)
  Saturation2/1 -> [Iqref]
  Sum4/1 -> Gain1/1
  [V_RMS] -> Sum4/2
  K_FRT/1 -> Saturation1/1
  Saturation1/1 -> Divide2/1
  Equal/1 -> Data Type Conversion/1
  Data Type Conversion/1 -> Divide2/2
  [vd] -> Equal/1
  Divide2/1 -> Add/1
  Constant12/1 -> Sum4/3
  Constant8/1 -> Sum4/1
  Constant9/1 -> Equal/2
  Constant4/1 -> Switch/2
  Add/1 -> Saturation2/1
  [Iqref_PI] -> Add/2
  Mux2/1 -> Inner Current Control/5(idq_max)
  Constant5/1 -> Mux2/2
  [Idmax] -> Mux2/1
  From16/1 -> LPF2/1(In1)
  Q_set/1 -> [Q_set]
  LPF1/1(Ref) -> PI_fw_init2/1
  Square1/1 -> Sum3/2
  Sqrt/1 -> [Idmax]
  Sum3/1 -> Sqrt/1
  Constant3/1 -> Square/1
  Square/1 -> Sum3/1
  [Iqref] -> Square1/1
  Gain1/1 -> K_FRT/1
  Sum5/1 -> Mux3/1
  From28/1 -> Gain3/1
  Demux2/2 -> Sum6/1
  Gain3/1 -> Demux2/1
  Constant2/1 -> Gain4/1
  norm1/1(Out1) -> Goto18/1
  Divide1/1 -> Sum5/3
  Sum6/1 -> Mux3/2
  Mux3/1 -> norm1/1(In1)
  Divide/1 -> Sum6/3
  Divide5/1 -> Divide/2, Divide1/2
  Demux2/1 -> Sum5/1
  Divide3/1 -> Sum5/2
  Demux3/2 -> Divide1/1, Divide4/1
  Divide4/1 -> Sum6/2
  Demux3/1 -> Divide/1, Divide3/1
  PLL/1(Theta_rad) -> [Theta_PLL]
  PLL/2(CosSinTheta) -> [CosSinTheta]
  PLL/3(w_pu) -> [w_PLL]
  From15/1 -> Divide5/2
  Constant7/1 -> Gain5/1
  From41/1 -> LPF1/1(In1)
  [vg_abc_pu] -> PLL/1(abc_pu)
  [vg_abc_pu] -> " pu P/Q computation"/1(v_abc_pu)
  [ig_abc_pu] -> " pu P/Q computation"/2(i_abc_pu)
  [ig_abc_pu] -> abc2dq0_norm/1
  [vm_dq] -> RMS derivation1/1(dq), Bus Generator1/2  "vm_dq"
  [vm_abc_ref_pu] -> vm_abc_ref_pu/1
  [vm_abc_ref_pu] -> Bus Generator1/1
  [vgdq] -> Inner Current Control/4(vg_dq)
  From39/1 -> PI_fw_init/2
  From29/1 -> Gain2/1
  Gain2/1 -> Demux3/1
  Gain5/1 -> Divide5/1
  Gain4/1 -> Divide4/2, Divide3/2
  From40/1 -> norm2/1(In1)
  norm2/1(Out1) -> Goto23/1
  PLL/4(vdq) -> Demux/1, [vgdq]
  Demux/1 -> [vd]
  Demux/2 -> [vq]
  [vgdq] -> RMS derivation/1(dq), Bus Generator/2
  RMS derivation/1(rms) -> Scope/1, [Vg_rms], Bus Generator/3  "Vg_RMS"
  [Theta_PLL] -> Bus Creator/4  "Theta"
  CosSin_Delay/1 -> dq02abc_norm/3
  LPF3/1(Out1) -> [V_RMS]
  [Vg_rms] -> LPF3/1(In1)
  Constant13/1 -> PI_fw_init1/4
  Constant14/1 -> PI_fw_init1/5
  PI_fw_init2/1 -> Switch/3
  Constant6/1 -> PI_fw_init2/2
  [w_PLL] -> Inner Current Control/3(w)
  Add18/1 -> [V_ref]
  Add17/1 -> Gain11/1
  Gain11/1 -> Add18/2
  [Q_set] -> Add17/1
  Constant26/1 -> Add18/1
  [Q] -> Add17/2
  [V_ref] -> Add1/1
  LPF7/1(Out1) -> Add1/2
  Constant16/1 -> PID Controller1/2, Gain/1
  Constant25/1 -> Divide8/2, Divide9/1
  Add1/1 -> Divide9/2
  Divide9/1 -> PID Controller3/1
  Divide8/1 -> PID Controller2/1
  Add6/1 -> Divide8/1
  PID Controller1/1 -> [Idref_PI]
  LPF6/1(Out1) -> Add6/2
  [P] -> LPF4/1(In1)
  LPF4/1(Out1) -> Add5/2
  Add5/1 -> PID Controller1/1
  Constant17/1 -> Switch1/2
  [Q] -> LPF6/1(In1)
  PID Controller2/1 -> Switch1/1
  [Vg_rms] -> LPF7/1(In1)
  PID Controller3/1 -> Switch1/3
  Gain/1 -> PID Controller1/3
  Switch1/1 -> [Iqref_PI]
  [P_set] -> Add5/1
  [Q_set] -> Add6/1
  Low-Pass Filter (Discrete or Continuous)1/1 -> [igdq], Scope3/1  "ig_dq"

== system benchmark_16bus_base_scenario/GFL IDEAL VSC8/Bridge_Model ==
  Uref : Inport
  NOT1 : Logic  Operator=NOT  IconShape=distinctive  AllPortsSameDT=off  OutDataTypeStr=boolean
  Saturation : Saturate  UpperLimit=1  LowerLimit=-1
  Step : Step  Time=Output_Delay  SampleTime=0
  Terminator : Terminator
  Three-Phase Breaker2 : spsThreePhaseBreakerLib/Three-Phase Breaker  InitialState=open  SwitchA=on  SwitchB=on  SwitchC=on  SwitchTimes="[4/60  10/60]"  External=on  BreakerResistance=1e-5*Zb  SnubberResistance=1e6  SnubberCapacitance=inf  Measurements=None
  Three-Phase Breaker3 : spsThreePhaseBreakerLib/Three-Phase Breaker  InitialState=closed  SwitchA=on  SwitchB=on  SwitchC=on  SwitchTimes="[4/60  10/60]"  External=on  BreakerResistance=1e-6*Zb  SnubberResistance=1e6  SnubberCapacitance=inf  Measurements=None
  Three-Phase Source : spsThreePhaseSourceLib/Three-Phase Source  InternalConnection=Yg  VoltagePhases=off  Voltage=Vm0*Un1  PhaseAngle=Theta_Vm0  Voltage_phases=[25e3 25e3 25e3]/sqrt(3)  PhaseAngles_phases=[0 -120 +120]  Frequency=fb  NonIdealSource=off  SpecifyImpedance=off  Resistance=0  Inductance=0  ShortCircuitLevel=100e6  BaseVoltage=VSC01_Un1  XRratio=7  BusType=swing  Pref=0.3  Qref=0  Prefabc=[10e3, 10e3, 10e3]  Qrefabc=[0, 0, 0]  Qmin=-Inf  Qmax=Inf
  Universal Bridge : spsUniversalBridgeLib/Universal Bridge  Arms=3  SnubberResistance=1e5  SnubberCapacitance=inf  Device=Average-model based VSC  Ron=1e-3  Lon=0  ForwardVoltages="[  0  0  ]"  ForwardVoltage=0  GTOparameters=[ 10e-6 , 20e-6 ]  IGBTparameters=[ 1e-6 , 2e-6 ]  Measurements=None  Measurements_2=None  converterType=Rectifier
  Vdc : spsVoltageMeasurementLib/Voltage Measurement  PhasorSimulation=off  OutputType=Complex  PSBequivalent=0
  mp3 : Gain  Gain=2/Udcn
  PhA : PMIOPort  Side=Right
  PhB : PMIOPort  Port=2  Side=Right
  PhC : PMIOPort  Port=3  Side=Right
  Vdc+ : PMIOPort  Port=4  Side=Left
  Vdc- : PMIOPort  Port=5  Side=Left
  wires:
  Step/1 -> Three-Phase Breaker2/1, NOT1/1
  Saturation/1 -> Universal Bridge/1
  NOT1/1 -> Three-Phase Breaker3/1
  mp3/1 -> Saturation/1
  Uref/1 -> mp3/1
  Vdc/1 -> Terminator/1
  connections:
  Three-Phase Breaker3/RConn3 -- Three-Phase Source/RConn3
  Three-Phase Breaker3/RConn2 -- Three-Phase Source/RConn2
  Three-Phase Breaker3/RConn1 -- Three-Phase Source/RConn1
  Three-Phase Breaker2/RConn1 -- Universal Bridge/LConn1
  Three-Phase Breaker2/RConn2 -- Universal Bridge/LConn2
  Three-Phase Breaker2/RConn3 -- Universal Bridge/LConn3
  Three-Phase Breaker2/LConn1 -- Three-Phase Breaker3/LConn1 -- PhA/RConn1
  Three-Phase Breaker2/LConn2 -- Three-Phase Breaker3/LConn2 -- PhB/RConn1
  Three-Phase Breaker2/LConn3 -- Three-Phase Breaker3/LConn3 -- PhC/RConn1
  Vdc/LConn1 -- Universal Bridge/RConn1 -- Vdc+/RConn1
  Vdc/LConn2 -- Universal Bridge/RConn2 -- Vdc-/RConn1
